simulink model "NonLinearActuator"  (Simulink 8.5)
settings: Solver=ode45  StartTime=0.0  StopTime=10.0  MaxStep=0.1  RelTol=1e-3
undefined symbols (not defined in the file): Ta
settings Model: Creator=The MathWorks Inc.  ModifiedByFormat=The MathWorks Inc.  LastModifiedBy=The MathWorks Inc.  CovSFcnEnable=off
settings DataIOCC: SignalLoggingSaveFormat=Dataset  SaveOutput=off  SaveTime=off  SignalLoggingName=NonLinearActuator
settings OptimizationCC: InlineParams=on  InitFltsAndDblsToZero=on  SimCompilerOptimization=Off
settings DebuggingCC: SaveWithParameterizedLinksMsg=none  SignalResolutionControl=TryResolveAllWithWarning  SolverPrmCheckMsg=warning  MultiTaskDSMMsg=warning  MultiTaskCondExecSysMsg=none  FcnCallInpInsideContextMsg=UseLocalSettings
settings ModelReferenceCC: ModelReferenceMinAlgLoopOccurrences=on
settings RTWCC: RTWCompilerOptimization=Off
settings GRTTargetCC: TargetFcnLib=ansi_tfl_tmw.mat

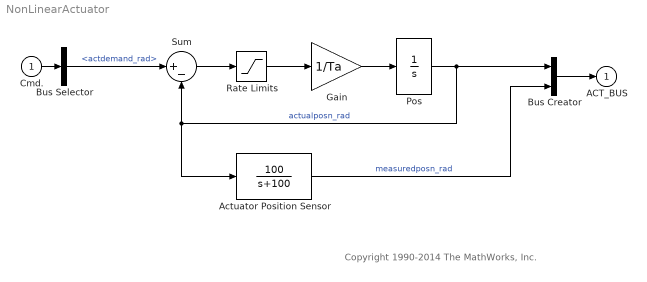
== system NonLinearActuator ==
  note: Copyright 1990-2014 The MathWorks, Inc.
  Cmd. : Inport  IOType=none  Commented=off  StatePerturbationForJacobian=1.0e-05  OutDataTypeStr=Bus: CONTROL_BUS
  Actuator Position Sensor : TransferFcn  IOType=none  Commented=off  StatePerturbationForJacobian=1.0e-05  Numerator=[100]  Denominator=[1 100]
  Bus Creator : BusCreator  IOType=none  Commented=off  StatePerturbationForJacobian=1.0e-05  Inputs=2  OutDataTypeStr=Bus: ACT_BUS
  Bus Selector : BusSelector  IOType=none  Commented=off  StatePerturbationForJacobian=1.0e-05  OutputSignals=actdemand_rad
  Gain : Gain  IOType=none  Commented=off  StatePerturbationForJacobian=1.0e-05  Gain=1/Ta  SaturateOnIntegerOverflow=on  OutDataTypeStr=Inherit: Same as input  ParamDataTypeStr=Inherit: Same as input
  Pos : Integrator  IOType=none  Commented=off  StatePerturbationForJacobian=1.0e-05  LimitOutput=on  UpperSaturationLimit=pi*45/180  LowerSaturationLimit=-pi*45/180
  Rate Limits : Saturate  IOType=none  Commented=off  StatePerturbationForJacobian=1.0e-05
  Sum : Sum  IOType=none  Commented=off  StatePerturbationForJacobian=1.0e-05  Inputs=|+-  SaturateOnIntegerOverflow=on  InputSameDT=on  OutDataTypeStr=Inherit: Same as first input
  ACT_BUS : Outport  IOType=none  Commented=off  StatePerturbationForJacobian=1.0e-05  OutDataTypeStr=Bus: ACT_BUS  InitialOutput=0  BusOutputAsStruct=on
  wires:
  Actuator Position Sensor/1 -> Bus Creator/2  "measuredposn_rad"
  Pos/1 -> Actuator Position Sensor/1, Sum/2, Bus Creator/1  "actualposn_rad"
  Sum/1 -> Rate Limits/1
  Gain/1 -> Pos/1
  Rate Limits/1 -> Gain/1
  Bus Creator/1 -> ACT_BUS/1
  Cmd./1 -> Bus Selector/1
  Bus Selector/1 -> Sum/1  "<actdemand_rad>"
